simulink model "PMSM_Progress_Model"  (R2023b)
settings: Solver=ode4  StartTime=0.0  StopTime=2  FixedStep=1e-4  RelTol=1e-3
values from neighbouring files (symbols this model uses):
  Ki = BW*rs    (= 12.5663706144)    [PI_parameters_STEADY_STATE_ROTOR_REFERANCED_PMSM.m]
  Kp = BW*Lq    (= 0.0188495559215)    [PI_parameters_STEADY_STATE_ROTOR_REFERANCED_PMSM.m]
libraries: slpidlib x2
settings Model: Creator=szymo  LastModifiedBy=szymo

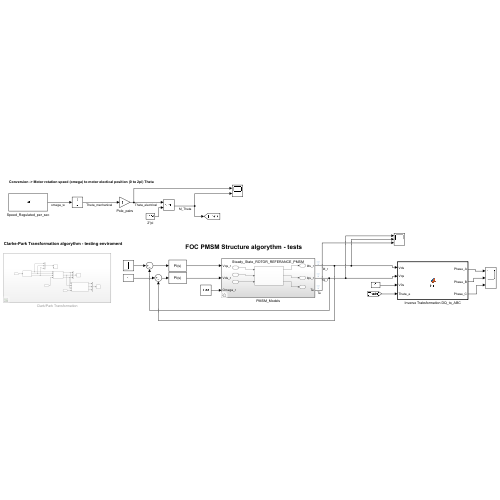
[thumbnail: Simulink's stored preview of the top-level diagram]
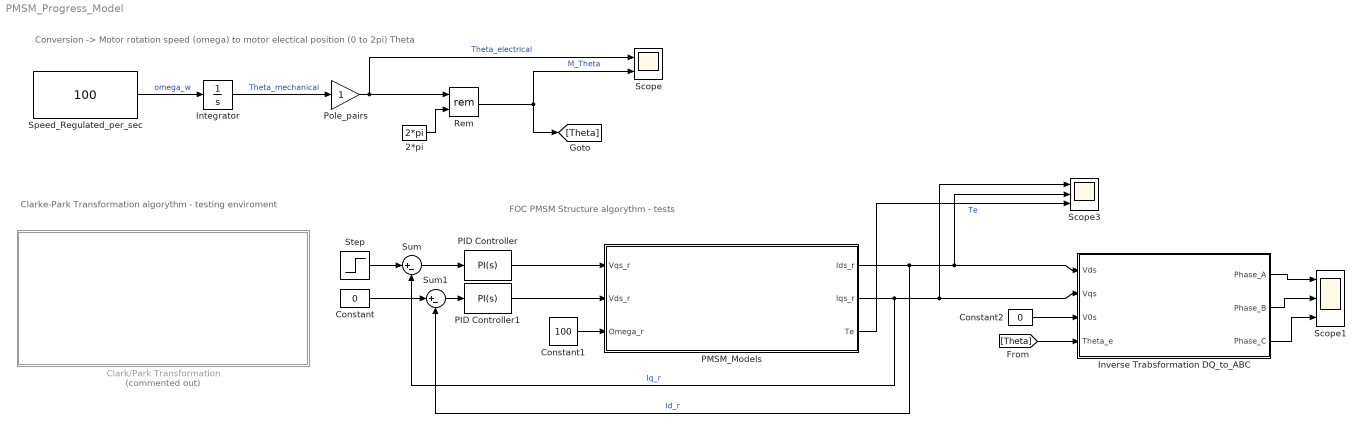
== system PMSM_Progress_Model ==
  note: FOC PMSM Structure algorythm - tests
  note: Clarke-Park Transformation algorythm - testing enviroment
  note: Conversion -> Motor rotation speed (omega) to motor electical position (0 to 2pi) Theta
  2*pi : Constant  Value=2*pi
  Clark/Park Transformation : Subsystem  Commented=on
  Constant : Constant  Value=0
  Constant1 : Constant  Value=100
  Constant2 : Constant  Value=0
  Integrator : Integrator
  Inverse Trabsformation DQ_to_ABC : MATLAB Function  TreatAsAtomicUnit=on
  PID Controller : slpidlib/PID Controller  Controller=PI  Form=Parallel  TimeDomain=Continuous-time  UseExternalTs=off  SampleTime=-1  IntegratorMethod=Forward Euler  FilterMethod=Forward Euler  ControllerParametersSource=internal  P=Kp  I=Ki  UseKiTs=off  D=0  N=100  UseFilter=on  TunerSelectOption=Transfer Function Based (PID Tuner App)  InitialConditionSource=internal  InitialConditionForIntegrator=0  InitialConditionForFilter=0  DifferentiatorICPrevScaledInput=0  ExternalReset=none  TrackingMode=off  Kt=1  LimitOutput=off  SatLimitsSource=internal  UpperSaturationLimit=inf  LowerSaturationLimit=-inf  LinearizeAsGain=on  AntiWindupMode=none  Kb=1  LimitIntegrator=off  UpperIntegratorSaturationLimit=inf  LowerIntegratorSaturationLimit=-inf  POutMin=[]  POutMax=[]  IOutMin=[]  IOutMax=[]  DOutMin=[]  DOutMax=[]  NOutMin=[]  NOutMax=[]  SumOutMin=[]  SumOutMax=[]  SaturationOutMin=[]  SaturationOutMax=[]  PParamMin=[]  PParamMax=[]  IParamMin=[]  IParamMax=[]  DParamMin=[]  DParamMax=[]  NParamMin=[]  NParamMax=[]  KbParamMin=[]  KbParamMax=[]  KtParamMin=[]  KtParamMax=[]  KbOutMin=[]  KbOutMax=[]  KtOutMin=[]  KtOutMax=[]  IntegratorOutMin=[]  IntegratorOutMax=[]  FilterOutMin=[]  FilterOutMax=[]  SumI1OutMin=[]  SumI1OutMax=[]  SumI2OutMin=[]  SumI2OutMax=[]  SumI3OutMin=[]  SumI3OutMax=[]  SumI4OutMin=[]  SumI4OutMax=[]  SumDOutMin=[]  SumDOutMax=[]  DifferentiatorOutMin=[]  DifferentiatorOutMax=[]  FilterDiffOutCoefMin=[]  FilterDiffOutCoefMax=[]  ReciprocalOutMin=[]  ReciprocalOutMax=[]  SumDenOutMin=[]  SumDenOutMax=[]  SumNumOutMin=[]  SumNumOutMax=[]  DivideOutMin=[]  DivideOutMax=[]  UdiffTsProdOutMin=[]  UdiffTsProdOutMax=[]  NTsProdOutMin=[]  NTsProdOutMax=[]  UintegralTsProdOutMin=[]  UintegralTsProdOutMax=[]  UngainTsProdOutMin=[]  UngainTsProdOutMax=[]  ClampingZeroOutDataTypeStr=Inherit: Inherit via back propagation  ClampingZeroOutMin=[]  ClampingZeroOutMax=[]  FilterDenConstantOutDataTypeStr=Inherit: Inherit via back propagation  FilterDenConstantOutMin=[]  FilterDenConstantOutMax=[]  PCopyOutDataTypeStr=Inherit: Inherit via back propagation  PCopyOutMin=[]  PCopyOutMax=[]  NCopyOutDataTypeStr=Inherit: Inherit via back propagation  NCopyOutMin=[]  NCopyOutMax=[]  IntegratorContinuousStateAttributes=''  IntegratorStateMustResolveToSignalObject=off  IntegratorRTWStateStorageClass=Auto  FilterContinuousStateAttributes=''  FilterStateMustResolveToSignalObject=off  FilterRTWStateStorageClass=Auto  ParallelPVariant=InternalParameters  IdealPVariant=Disabled  IVariant=InternalParameters  DVariant=Disabled  IntegratorVariant=Continuous  SatVariant=Disabled  AWVariant=Passthrough  PCopyVariant=Disabled  TRVariant=Disabled  FdbkBlocksVariant=Forward  IdealPFdbkVariant=Disabled  SatFdbkVariant=Disabled  DerivativeFilterVariant=Disabled  NVariant=Disabled  NCopyVariant=Disabled_SignalSpec  FilterICVariant=Disabled  IntegratorICVariant=InternalICs  ExternalResetVariant=Disabled  TRSumVariant=Passthrough  SumFdbkVariant=Disabled  SumVariant=Sum_PI  TsampFilterVariant=InternalTs  TsampNgainVariant=Passthrough  TsampIntegralVariant=Disabled_SignalSpec  ExternalSaturationOutDataTypeStr=Inherit: Same as second input
  PID Controller1 : slpidlib/PID Controller  Controller=PI  Form=Parallel  TimeDomain=Continuous-time  UseExternalTs=off  SampleTime=-1  IntegratorMethod=Forward Euler  FilterMethod=Forward Euler  ControllerParametersSource=internal  P=Kp  I=Ki  UseKiTs=off  D=0  N=100  UseFilter=on  TunerSelectOption=Transfer Function Based (PID Tuner App)  InitialConditionSource=internal  InitialConditionForIntegrator=0  InitialConditionForFilter=0  DifferentiatorICPrevScaledInput=0  ExternalReset=none  TrackingMode=off  Kt=1  LimitOutput=off  SatLimitsSource=internal  UpperSaturationLimit=inf  LowerSaturationLimit=-inf  LinearizeAsGain=on  AntiWindupMode=none  Kb=1  LimitIntegrator=off  UpperIntegratorSaturationLimit=inf  LowerIntegratorSaturationLimit=-inf  POutMin=[]  POutMax=[]  IOutMin=[]  IOutMax=[]  DOutMin=[]  DOutMax=[]  NOutMin=[]  NOutMax=[]  SumOutMin=[]  SumOutMax=[]  SaturationOutMin=[]  SaturationOutMax=[]  PParamMin=[]  PParamMax=[]  IParamMin=[]  IParamMax=[]  DParamMin=[]  DParamMax=[]  NParamMin=[]  NParamMax=[]  KbParamMin=[]  KbParamMax=[]  KtParamMin=[]  KtParamMax=[]  KbOutMin=[]  KbOutMax=[]  KtOutMin=[]  KtOutMax=[]  IntegratorOutMin=[]  IntegratorOutMax=[]  FilterOutMin=[]  FilterOutMax=[]  SumI1OutMin=[]  SumI1OutMax=[]  SumI2OutMin=[]  SumI2OutMax=[]  SumI3OutMin=[]  SumI3OutMax=[]  SumI4OutMin=[]  SumI4OutMax=[]  SumDOutMin=[]  SumDOutMax=[]  DifferentiatorOutMin=[]  DifferentiatorOutMax=[]  FilterDiffOutCoefMin=[]  FilterDiffOutCoefMax=[]  ReciprocalOutMin=[]  ReciprocalOutMax=[]  SumDenOutMin=[]  SumDenOutMax=[]  SumNumOutMin=[]  SumNumOutMax=[]  DivideOutMin=[]  DivideOutMax=[]  UdiffTsProdOutMin=[]  UdiffTsProdOutMax=[]  NTsProdOutMin=[]  NTsProdOutMax=[]  UintegralTsProdOutMin=[]  UintegralTsProdOutMax=[]  UngainTsProdOutMin=[]  UngainTsProdOutMax=[]  ClampingZeroOutDataTypeStr=Inherit: Inherit via back propagation  ClampingZeroOutMin=[]  ClampingZeroOutMax=[]  FilterDenConstantOutDataTypeStr=Inherit: Inherit via back propagation  FilterDenConstantOutMin=[]  FilterDenConstantOutMax=[]  PCopyOutDataTypeStr=Inherit: Inherit via back propagation  PCopyOutMin=[]  PCopyOutMax=[]  NCopyOutDataTypeStr=Inherit: Inherit via back propagation  NCopyOutMin=[]  NCopyOutMax=[]  IntegratorContinuousStateAttributes=''  IntegratorStateMustResolveToSignalObject=off  IntegratorRTWStateStorageClass=Auto  FilterContinuousStateAttributes=''  FilterStateMustResolveToSignalObject=off  FilterRTWStateStorageClass=Auto  ParallelPVariant=InternalParameters  IdealPVariant=Disabled  IVariant=InternalParameters  DVariant=Disabled  IntegratorVariant=Continuous  SatVariant=Disabled  AWVariant=Passthrough  PCopyVariant=Disabled  TRVariant=Disabled  FdbkBlocksVariant=Forward  IdealPFdbkVariant=Disabled  SatFdbkVariant=Disabled  DerivativeFilterVariant=Disabled  NVariant=Disabled  NCopyVariant=Disabled_SignalSpec  FilterICVariant=Disabled  IntegratorICVariant=InternalICs  ExternalResetVariant=Disabled  TRSumVariant=Passthrough  SumFdbkVariant=Disabled  SumVariant=Sum_PI  TsampFilterVariant=InternalTs  TsampNgainVariant=Passthrough  TsampIntegralVariant=Disabled_SignalSpec  ExternalSaturationOutDataTypeStr=Inherit: Same as second input
  PMSM_Models : Subsystem  Variant=on
  Pole_pairs : Gain
  Rem : Math  Operator=rem
  Scope : Scope  NumInputPorts=2
  Scope1 : Scope  NumInputPorts=3
  Scope3 : Scope  NumInputPorts=3
  Speed_Regulated_per_sec : Constant  Value=100
  Step : Step  After=2  SampleTime=0
  Sum : Sum  Inputs=|+-
  Sum1 : Sum  Inputs=|+-
  wires:
  Speed_Regulated_per_sec/1 -> Integrator/1  "omega_w"
  Integrator/1 -> Pole_pairs/1  "Theta_mechanical"
  Pole_pairs/1 -> Rem/1, Scope/1  "Theta_electrical"
  2*pi/1 -> Rem/2
  Rem/1 -> [Theta], Scope/2  "M_Theta"
  Constant1/1 -> PMSM_Models/3(Omega_r)
  PMSM_Models/1(Ids_r) -> Sum1/2, Scope3/2, Inverse Trabsformation DQ_to_ABC/1(Vds)  "Id_r"
  PMSM_Models/2(Iqs_r) -> Sum/2, Scope3/1, Inverse Trabsformation DQ_to_ABC/2(Vqs)  "Iq_r"
  Constant2/1 -> Inverse Trabsformation DQ_to_ABC/3(V0s)
  [Theta] -> Inverse Trabsformation DQ_to_ABC/4(Theta_e)
  Inverse Trabsformation DQ_to_ABC/1(Phase_A) -> Scope1/1
  Inverse Trabsformation DQ_to_ABC/2(Phase_B) -> Scope1/2
  Inverse Trabsformation DQ_to_ABC/3(Phase_C) -> Scope1/3
  PID Controller/1 -> PMSM_Models/1(Vqs_r)
  PID Controller1/1 -> PMSM_Models/2(Vds_r)
  Step/1 -> Sum/1
  Sum/1 -> PID Controller/1
  Sum1/1 -> PID Controller1/1
  Constant/1 -> Sum1/1
  PMSM_Models/3(Te) -> Scope3/3  "Te"

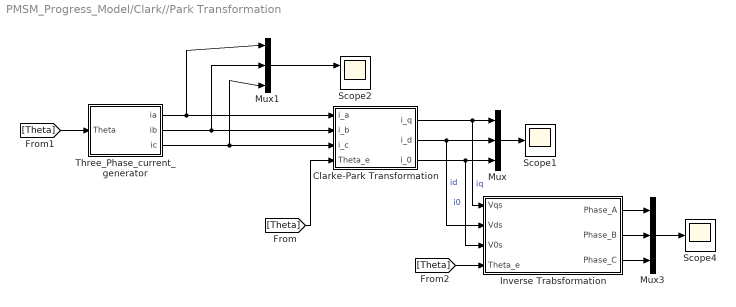
== system PMSM_Progress_Model/Clark//Park Transformation ==
  Clarke-Park Transformation : MATLAB Function  TreatAsAtomicUnit=on
  Inverse Trabsformation : MATLAB Function  TreatAsAtomicUnit=on
  Mux : Mux  Inputs=3
  Mux1 : Mux  Inputs=3
  Mux3 : Mux  Inputs=3
  Scope1 : Scope
  Scope2 : Scope  NumInputPorts=2
  Scope4 : Scope
  Three_Phase_current_generator : MATLAB Function  TreatAsAtomicUnit=on
  wires:
  Clarke-Park Transformation/1(i_q) -> Inverse Trabsformation/1(Vqs), Mux/1  "iq"
  [Theta] -> Clarke-Park Transformation/4(Theta_e)
  Three_Phase_current_generator/1(ia) -> Mux1/1, Clarke-Park Transformation/1(i_a)
  Clarke-Park Transformation/2(i_d) -> Inverse Trabsformation/2(Vds), Mux/2  "id"
  Three_Phase_current_generator/3(ic) -> Mux1/3, Clarke-Park Transformation/3(i_c)
  Inverse Trabsformation/3(Phase_C) -> Mux3/3
  Mux3/1 -> Scope4/1
  Clarke-Park Transformation/3(i_0) -> Inverse Trabsformation/3(V0s), Mux/3  "i0"
  [Theta] -> Three_Phase_current_generator/1(Theta)
  Mux1/1 -> Scope2/1
  Inverse Trabsformation/1(Phase_A) -> Mux3/1
  Inverse Trabsformation/2(Phase_B) -> Mux3/2
  Three_Phase_current_generator/2(ib) -> Mux1/2, Clarke-Park Transformation/2(i_b)
  [Theta] -> Inverse Trabsformation/4(Theta_e)
  Mux/1 -> Scope1/1

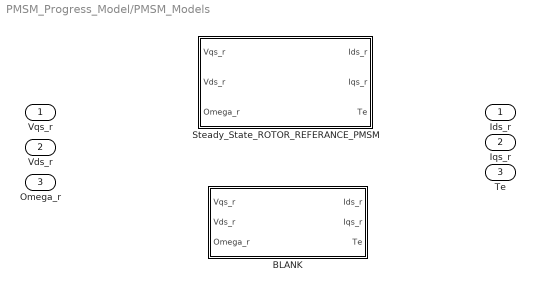
== system PMSM_Progress_Model/PMSM_Models ==
  Vqs_r : Inport
  Vds_r : Inport  Port=2
  Omega_r : Inport  Port=3
  BLANK : Subsystem  VariantControl=Model==2
  Steady_State_ROTOR_REFERANCE_PMSM : Subsystem  VariantControl=Model==1
  Ids_r : Outport
  Iqs_r : Outport  Port=2
  Te : Outport  Port=3

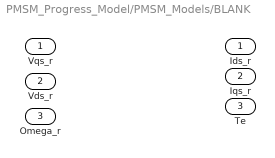
== system PMSM_Progress_Model/PMSM_Models/BLANK ==
  Vqs_r : Inport
  Vds_r : Inport  Port=2
  Omega_r : Inport  Port=3
  Ids_r : Outport
  Iqs_r : Outport  Port=2
  Te : Outport  Port=3

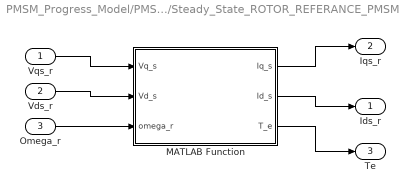
== system PMSM_Progress_Model/PMSM_Models/Steady_State_ROTOR_REFERANCE_PMSM ==
  Vqs_r : Inport
  Vds_r : Inport  Port=2
  Omega_r : Inport  Port=3
  MATLAB Function : MATLAB Function  TreatAsAtomicUnit=on
  Ids_r : Outport
  Iqs_r : Outport  Port=2
  Te : Outport  Port=3
  wires:
  Vqs_r/1 -> MATLAB Function/1(Vq_s)
  Vds_r/1 -> MATLAB Function/2(Vd_s)
  Omega_r/1 -> MATLAB Function/3(omega_r)
  MATLAB Function/3(T_e) -> Te/1
  MATLAB Function/1(Iq_s) -> Iqs_r/1
  MATLAB Function/2(Id_s) -> Ids_r/1

== matlab function PMSM_Progress_Model/Clark//Park Transformation/Three_Phase_current_generator ==
  data: Theta input; ia output; ib output; ic output
function [ia,ib,ic] = fcn(Theta)

ia = cos(Theta);
ib = cos(Theta - (2*pi/3));
ic= cos(Theta + (2*pi/3));

end

== matlab function PMSM_Progress_Model/Clark//Park Transformation/Clarke-Park Transformation ==
  data: i_a input; i_q output; i_b input; i_c input; Theta_e input; i_d output; i_0 output
function [i_q, i_d, i_0] = fcn(i_a, i_b, i_c, Theta_e)

% The transform matrix

% Ks = (2/3) * [cos(Theta_e) cos(Theta_e-(2*pi/3)) cos(Theta_e+(2*pi/3))
%               sin(Theta_e) sin(Theta_e-(2*pi/3)) sin(Theta_e+(2*pi/3))
%               0.5          0.5                   0.5                 ]  
%
% [i_q; 
% i_d; = Ks*[i_a, i_b, i_c]
% i_0]

i_q = (2/3)*(cos(Theta_e)*i_a + cos(Theta_e-(2*pi/3))*i_b + cos(Theta_e+(2*pi/3))*i_c);
i_d = (2/3)*(sin(Theta_e)*i_a + sin(Theta_e-(2*pi/3))*i_b + sin(Theta_e+(2*pi/3))*i_c);
i_0 = (2/3)*0.5*(i_a+i_b+i_c);



end

== matlab function PMSM_Progress_Model/Clark//Park Transformation/Inverse Trabsformation ==
  data: Phase_A output; Phase_B output; Phase_C output; Vqs input; Vds input; V0s input; Theta_e input
function [Phase_A, Phase_B, Phase_C] = fcn(Vqs, Vds, V0s, Theta_e)

%Inverse function od Iq and Id (DC signals) to three phase A, B and C 
%signals later used for controlling PMSM

%Rotor electrical position
Theta=Theta_e;

%Phase equations
Phase_A = cos(Theta)*Vqs + sin(Theta)*Vds + V0s*1;
Phase_B = cos(Theta-(2*pi/3))*Vqs + sin(Theta-(2*pi/3))*Vds+V0s*1;
Phase_C = cos(Theta+(2*pi/3))*Vqs + sin(Theta+(2*pi/3))*Vds+V0s*1;

end

== matlab function PMSM_Progress_Model/PMSM_Models/Steady_State_ROTOR_REFERANCE_PMSM/MATLAB Function ==
  data: Vq_s input; Iq_s output; Id_s output; T_e output; Vd_s input; omega_r input
function [Iq_s, Id_s, T_e] = fcn(Vq_s, Vd_s, omega_r)

%Physical constans of the PMSM - steady state
rs = 0.2;
Lq = 300e-6;
Ld = 300e-6;
Lambda_m_r = 0.01;
P = 2; %Poles (one pole pair)


%Evaluation of DC currents for d and q axis and torque 
K1 = ((rs^2)+(omega_r^2)*Lq*Ld);

Iq_s = (rs/K1)*(Vq_s-omega_r*Lambda_m_r-(omega_r*Ld/rs)*Vd_s);
Id_s = (1/K1)*(rs*Vd_s+omega_r*Lq*Vq_s-(omega_r^2)*Lq*Lambda_m_r);

T_e = (3/2)*(P/2)*(Lambda_m_r*Iq_s+(Ld-Lq)*Iq_s*Id_s);

end

== matlab function PMSM_Progress_Model/Inverse Trabsformation DQ_to_ABC ==
  data: Phase_A output; Phase_B output; Phase_C output; Vds input; Vqs input; V0s input; Theta_e input
function [Phase_A, Phase_B, Phase_C] = fcn(Vds, Vqs, V0s, Theta_e)

%Inverse function od Iq and Id (DC signals) to three phase A, B and C 
%signals later used for controlling PMSM

%Rotor electrical position
Theta=Theta_e;

%Phase equations
Phase_A = cos(Theta)*Vqs + sin(Theta)*Vds + V0s*1;
Phase_B = cos(Theta-(2*pi/3))*Vqs + sin(Theta-(2*pi/3))*Vds+V0s*1;
Phase_C = cos(Theta+(2*pi/3))*Vqs + sin(Theta+(2*pi/3))*Vds+V0s*1;

end
